simulink model "SSiWD_Lab2_blocks"  (R2015a)
settings: Solver=ode45  StartTime=0.0  StopTime=13  FixedStep=0.001  RelTol=1e-3
undefined symbols (not defined in the file or in its folder): sigbuilder_block
libraries: simulink x3, fuzblock x1
settings Model: Creator=Wojtek  LastModifiedBy=Szwank
settings DataIOCC: SignalLoggingSaveFormat=ModelDataLogs
settings DebuggingCC: SaveWithParameterizedLinksMsg=none  UnderspecifiedInitializationDetection=Classic  MergeDetectMultiDrivingBlocksExec=none  SolverPrmCheckMsg=warning  MultiTaskCondExecSysMsg=none  FcnCallInpInsideContextMsg=EnableAllAsWarning
settings GRTTargetCC: GeneratePreprocessorConditionals=Use local settings  CombineOutputUpdateFcns=off  GRTInterface=on

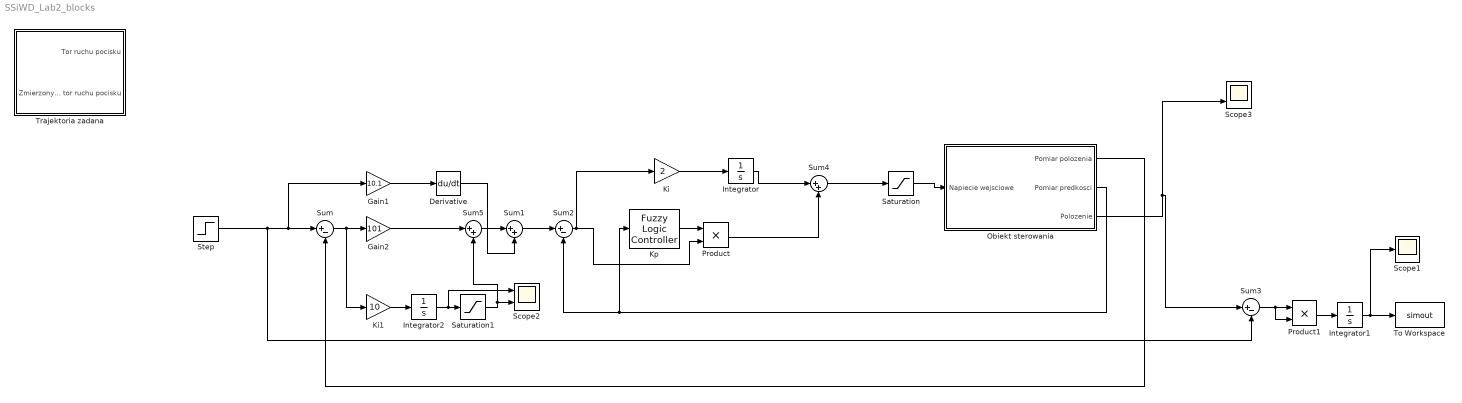
== system SSiWD_Lab2_blocks ==
  Derivative : Derivative
  Gain1 : Gain  Gain=10.1
  Gain2 : Gain  Gain=101
  Integrator : Integrator
  Integrator1 : Integrator  AbsoluteTolerance=0.001
  Integrator2 : Integrator
  Ki : Gain  Gain=2
  Ki1 : Gain  Gain=10
  Kp : fuzblock/Fuzzy Logic  Controller  fis=['regulator_prędkości.fis']
  Obiekt sterowania : Subsystem
  Product : Product
  Product1 : Product
  Saturation : Saturate  UpperLimit=50  LowerLimit=-50
  Saturation1 : Saturate  UpperLimit=70  LowerLimit=-70
  Scope1 : Scope
      settings: TimeRange=auto  MaxDataPoints=5000  SaveToWorkspace=off  YMin=-0.27846  YMax=2.50612  SampleTime=-1
  Scope2 : Scope  NumInputPorts=2
      settings: TimeRange=auto  MaxDataPoints=5000  SaveToWorkspace=off  SaveName=ScopeData2  YMin=-4.33652~-5  YMax=5.5637~5  SampleTime=-1
  Scope3 : Scope  NumInputPorts=2
      settings: TimeRange=auto  MaxDataPoints=5000  SaveToWorkspace=off  YMin=-1.96907~-5  YMax=4.71759~5  SampleTime=-1
  Step : Step  SampleTime=0.75
  Sum : Sum  Inputs=|+-
  Sum1 : Sum  Inputs=|++
  Sum2 : Sum  Inputs=|+-
  Sum3 : Sum  Inputs=|+-
  Sum4 : Sum  Inputs=|++
  Sum5 : Sum  Inputs=|++
  To Workspace : ToWorkspace  VariableName=simout  SampleTime=-1
  "Trajektoria zadana " : Subsystem
  wires:
  Obiekt sterowania/2(Pomiar predkosci) -> Kp/1, Sum2/2
  Obiekt sterowania/1(Pomiar polozenia) -> Sum/2
  Ki/1 -> Integrator/1
  Integrator/1 -> Sum4/1
  Saturation/1 -> Obiekt sterowania/1(Napiecie wejsciowe)
  Sum4/1 -> Saturation/1
  Product/1 -> Sum4/2
  Sum2/1 -> Ki/1, Product/2
  Derivative/1 -> Sum1/2
  Gain1/1 -> Derivative/1
  Kp/1 -> Product/1
  Integrator1/1 -> Scope1/1, To Workspace/1
  Sum/1 -> Ki1/1, Gain2/1
  Ki1/1 -> Integrator2/1
  Sum5/1 -> Sum1/1
  Gain2/1 -> Sum5/1
  Obiekt sterowania/3(Polozenie) -> Scope3/2, Sum3/1
  Sum1/1 -> Sum2/1
  Sum3/1 -> Product1/2, Product1/1
  Product1/1 -> Integrator1/1
  Integrator2/1 -> Scope2/1, Saturation1/1
  Saturation1/1 -> Scope2/2, Sum5/2
  Step/1 -> Sum3/2, Gain1/1, Sum/1

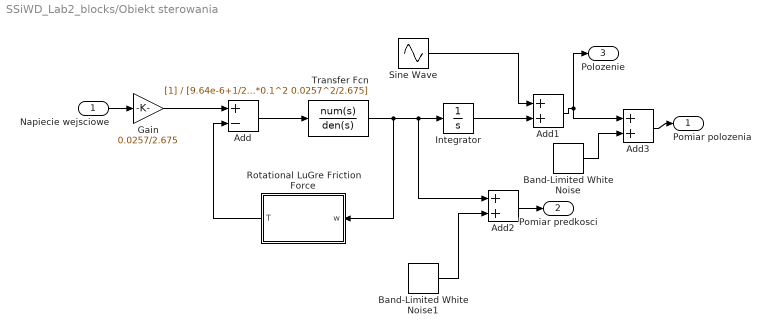
== system SSiWD_Lab2_blocks/Obiekt sterowania ==
  Napiecie wejsciowe : Inport
  Add : Sum  Inputs=+-
  Add1 : Sum
  Add2 : Sum
  Add3 : Sum
  Band-Limited White Noise : simulink/Sources/Band-Limited White Noise  Cov=[0.00001]  Ts=0.001  seed=[23341]
  Band-Limited White Noise1 : simulink/Sources/Band-Limited White Noise  Cov=[0.00001]  Ts=0.001  seed=[23341]
  Gain : Gain  Gain=0.0257/2.675
  Integrator : Integrator
  Rotational LuGre Friction Force : Subsystem  TreatAsAtomicUnit=on  mask(LuGre friction model){ro0=1.2, ro1=0.05, ro2=2.9e-6, Fc=0.77e-3, Fs=12e-3, Vs=0.09}
      mask prompts: Fc "Culomb force (Fc)"; Fs "Friction force (Fs)"; Vs "Striback velocity (Vs)"
      mask help:
      | The LuGre model is a dynamic friction model. The model is related to the bristle interpretation of friction. Friction is modeled as the average deflection force of elastic springs. When a tangential force is applied the bristles will deflect like springs. If the deflection is sufficiently large the bristles start to slip.
      |
      | The input signal is the velocity of the object. The output signal is the fristion force value.
      mask Help:
      | <!DOCTYPE html   PUBLIC "-//W3C//DTD HTML 4.01 Transitional//EN" "http://www.w3.org/TR/1999/REC-html401-19991224/loose.dtd">
      | <html lang="en"><head>
      | <meta http-equiv="Content-Type" content="text/html; charset=utf-8">
      | <title>About :: LuGre friction model</title>
      | <meta name="description" content="">
      | </head>
      | <body><a name="top_of_page"></a>
      | The LuGre model is a dynamic friction model. The model is related to
      | the bristle interpretation of friction. Friction is modeled as the average
      | deflection force of elastic springs. When a tangential force is applied the bristles
      | will deflect like springs. If the deflection is sufficiently large the bristles start
      | to slip. The average bristle deflection for a steady state motion is determined
      | by the velocity. It is lower at low velocities, which implies that the steady state
      | deflection decreases with increasing velocity. This models the phenomenon that
      | the surfaces are pushed apart by the lubricant, and models the Stribeck effect.
      | The model also includes rate dependent friction phenomena such as varying
      | break-away force and frictional lag.<sup><a href="#ref1">1</a></sup></p><p>More information about the model may be found in the labsheets.</p>
      | <hr><small>
      | <sup><a name="ref1"></a>1</sup> <b>Friction Models and Friction Compensation</b>. H. Olsson, K.J. &Aring;str&ouml;m, C. Canudas de Wit, M. G&auml;fvert, P. Lischinsky
      | </small>
      | <br />
      | <br />
      | <hr>
      | <center><small>Copyright&copy;2009
      | <a href="mailto:w.kurek@ely.pg.gda.pl">Wojciech Kurek</a>,
      | <a href="mailto:g.ewald@ely.pg.gda.pl">Grzegorz Ewald</a>
      | </small></center>
      | </body>
      | </html>
      mask Callback ro0:
      | if str2num(get_param(gcb, 'ro0')) <= 0
      |     error('ro0 is negative!')
      | end
      mask Callback ro1:
      | if str2num(get_param(gcb, 'ro1')) <= 0
      |     error('ro1 is negative!')
      | end
      mask Callback ro2:
      | if str2num(get_param(gcb, 'ro2')) <= 0
      |     error('ro2 is negative!')
      | end
      mask Callback Fc:
      | if str2num(get_param(gcb, 'Fs')) <= 0
      |     error('Culomb force is negative!')
      | end
      mask Callback Fs:
      | if str2num(get_param(gcb, 'Fs')) <= 0
      |     error('Friction force is negative!')
      | end
      mask Callback Vs:
      | if str2num(get_param(gcb, 'Vs')) <= 0
      |     error('Striback velocity is negative!')
      | end
      mask Display:
      | patch([0.1 0.1 0.9 0.9],[0.1 0.25 0.25 0.1],[0.8 0.8 0.8])
      | patch([0.1 0.1 0.9 0.9],[0.9 0.75 0.75 0.9],[0.8 0.8 0.8])
      | 
      | plot([0.12 0.12],[0.25 0.5])
      | plot([0.2 0.2],[0.25 0.5])
      | plot([0.4 0.4],[0.25 0.5])
      | plot([0.57 0.57],[0.25 0.5])
      | plot([0.67 0.67],[0.25 0.5])
      | plot([0.87 0.87],[0.25 0.5])
      | 
      | plot([0.17 0.18 0.2 0.23],[0.75 0.6 0.5 0.45])
      | plot([0.35 0.36 0.39 0.44],[0.75 0.6 0.5 0.48])
      | plot([0.62 0.64 0.68 0.72],[0.75 0.6 0.5 0.48])
      | plot([0.85 0.86 0.87 0.89],[0.75 0.6 0.5 0.48])
      | 
      | plot([0.15 0.15],[0.75 0.4])
      | plot([0.28 0.28],[0.75 0.4])
      | plot([0.55 0.55],[0.75 0.4])
      | plot([0.8 0.8],[0.75 0.4])
      | 
      | color('blue');
      | port_label('input',1,'\omega','texmode','on')
      | port_label('output',1,'T','texmode','on')
  Sine Wave : Sin  Amplitude=10  SampleTime=0
  Transfer Fcn : TransferFcn  Denominator=[9.64e-6+1/2*2.1*0.1^2 0.0257^2/2.675]
  Pomiar polozenia : Outport
  Pomiar predkosci : Outport  Port=2
  Polozenie : Outport  Port=3
  wires:
  Band-Limited White Noise/1 -> Add3/2
  Add3/1 -> Pomiar polozenia/1
  Add2/1 -> Pomiar predkosci/1
  Napiecie wejsciowe/1 -> Gain/1
  Add1/1 -> Add3/1, Polozenie/1
  Band-Limited White Noise1/1 -> Add2/2
  Integrator/1 -> Add1/2
  Sine Wave/1 -> Add1/1
  Add/1 -> Transfer Fcn/1
  Rotational LuGre Friction Force/1(T) -> Add/2
  Transfer Fcn/1 -> Add2/1, Integrator/1, Rotational LuGre Friction Force/1(w)
  Gain/1 -> Add/1

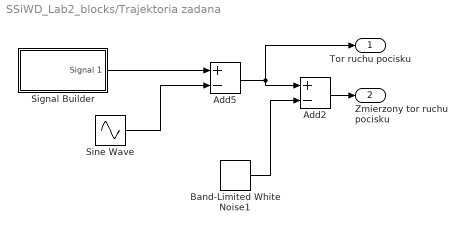
== system SSiWD_Lab2_blocks/Trajektoria zadana  ==
  Add2 : Sum  Inputs=+-
  Add5 : Sum  Inputs=+-
  Band-Limited White Noise1 : simulink/Sources/Band-Limited White Noise  Cov=[0.00001]  Ts=0.001  seed=[23341]
  Signal Builder : Subsystem  Tag=STV Subsys  LoadFcn=sigbuilder_block('load');  StartFcn=sigbuilder_block('start');  StopFcn=sigbuilder_block('stop');  ClipboardFcn=sigbuilder_block('clipboard');  mask(Sigbuilder block){}
      mask help: Simulink:masks:SigbuilderBlock_MD
      mask init:
      | if ~strcmp(get_param(bdroot(gcbh),'SimulationStatus'),'stopped') tuvar = sigbuilder_block('maskInit'); end
      settings: CopyFcn=sigbuilder_block('copy');  DeleteFcn=sigbuilder_block('delete');  ModelCloseFcn=sigbuilder_block('modelClose');  PreSaveFcn=sigbuilder_block('preSave');  PauseFcn=sigbuilder_block('pause');  ContinueFcn=sigbuilder_block('continue');  NameChangeFcn=sigbuilder_block('namechange');  OpenFcn=sigbuilder_block('open',[437.6 199.2 550.4 400 ]);  CloseFcn=sigbuilder_block('close');
      mask Display: plot(0, 0, 100, 100,[2, 2, 32, 32, 2], [68, 8, 8, 68, 68],[32, 2], [38, 38], [32, 19, 2],[53, 60, 44], [32, 17, 17, 2],[16, 16, 31, 31]);txt = getActiveGroup(gcbh);text(2, 100, txt,'verticalAlignment', 'top');
  Sine Wave : Sin  Amplitude=2  SampleTime=0
  Tor ruchu pocisku : Outport
  Zmierzony tor ruchu pocisku : Outport  Port=2
  wires:
  Add2/1 -> Zmierzony tor ruchu pocisku/1
  Sine Wave/1 -> Add5/2
  Signal Builder/1(Signal 1) -> Add5/1
  Add5/1 -> Tor ruchu pocisku/1, Add2/1
  Band-Limited White Noise1/1 -> Add2/2

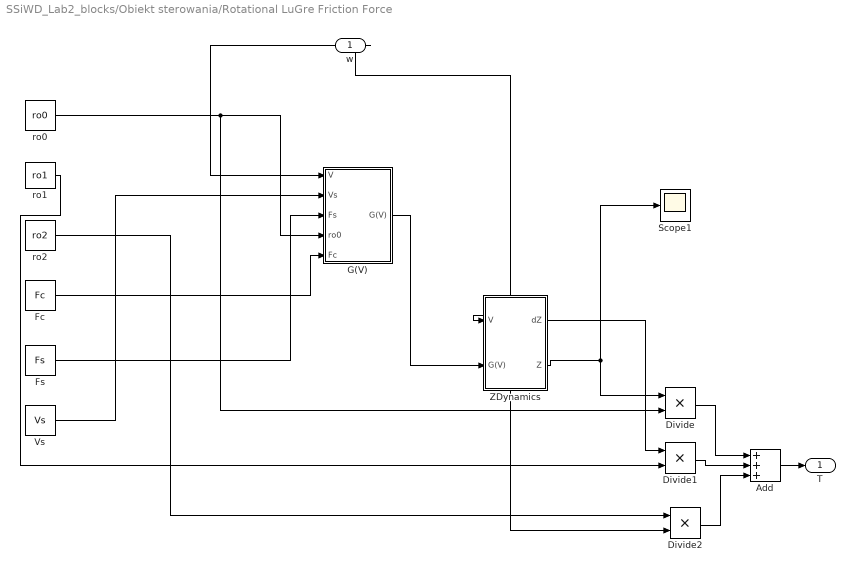
== system SSiWD_Lab2_blocks/Obiekt sterowania/Rotational LuGre Friction Force ==
  w : Inport
  Add : Sum  Inputs=+++
  Divide : Product  Inputs=**
  Divide1 : Product  Inputs=**
  Divide2 : Product  Inputs=**
  Fc : Constant  Value=Fc
  Fs : Constant  Value=Fs
  G(V) : Subsystem
  Scope1 : Scope
      settings: TimeRange=auto  MaxDataPoints=5000  SaveToWorkspace=off  SaveName=ScopeData3  YMin=-1  YMax=1  SampleTime=-1
  Vs : Constant  Value=Vs
  ZDynamics : Subsystem
  ro0 : Constant  Value=ro0
  ro1 : Constant  Value=ro1
  ro2 : Constant  Value=ro2
  T : Outport
  wires:
  Add/1 -> T/1
  Divide2/1 -> Add/3
  Divide1/1 -> Add/2
  Divide/1 -> Add/1
  ro2/1 -> Divide2/1
  ro1/1 -> Divide1/2
  ZDynamics/1(dZ) -> Divide1/1
  ZDynamics/2(Z) -> Scope1/1, Divide/1
  G(V)/1(G(V)) -> ZDynamics/2(G(V))
  ro0/1 -> Divide/2, G(V)/4(ro0)
  Fc/1 -> G(V)/5(Fc)
  Fs/1 -> G(V)/3(Fs)
  Vs/1 -> G(V)/2(Vs)
  w/1 -> G(V)/1(V), ZDynamics/1(V), Divide2/2

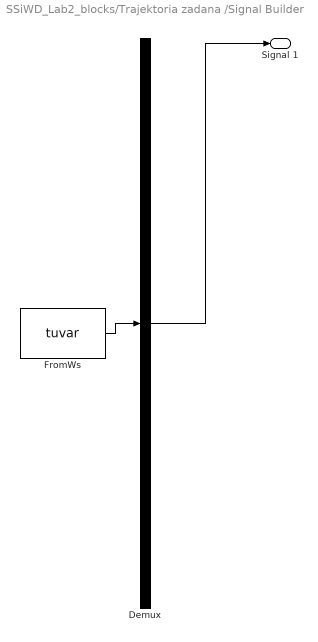
== system SSiWD_Lab2_blocks/Trajektoria zadana /Signal Builder ==
  Demux : Demux  Tag=STV Demux  Outputs=1
  FromWs : FromWorkspace  Tag=STV FromWs  VariableName=tuvar  SampleTime=0
      SigBuilderData=|
      | common.afterFinalStr = 'Extrapolate'
      | common.sampleTime = 0
      | dataSet.timeRange = [0 20]
      | dataSet.name = 'Group 1'
      | sbobj.Groups.Name = 'Group 1'
      | sbobj.Groups.Signals.Name = 'Signal 1'
      | sbobj.Groups.Signals.XData = [0 4 6 9 13.5 15.4 20]
      | sbobj.Groups.Signals.YData = [30 31 32 24 7 1.2 0]
      | sbobj.Groups.TimeRange = [0 20]
  Signal 1 : Outport  Tag=STV Outport
  wires:
  Demux/1 -> Signal 1/1
  FromWs/1 -> Demux/1

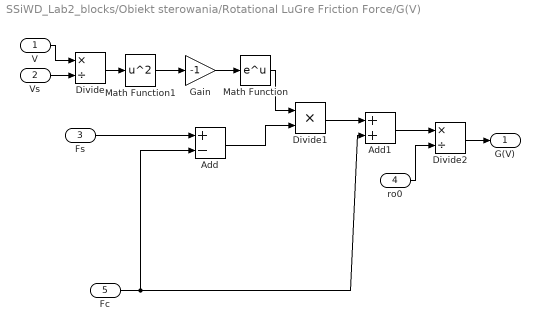
== system SSiWD_Lab2_blocks/Obiekt sterowania/Rotational LuGre Friction Force/G(V) ==
  V : Inport
  Vs : Inport  Port=2
  Fs : Inport  Port=3
  ro0 : Inport  Port=4
  Fc : Inport  Port=5
  Add : Sum  Inputs=+-
  Add1 : Sum
  Divide : Product  Inputs=*/
  Divide1 : Product  Inputs=**
  Divide2 : Product  Inputs=*/
  Gain : Gain  Gain=-1
  Math Function : Math  SaturateOnIntegerOverflow=on
  Math Function1 : Math  Operator=square  SaturateOnIntegerOverflow=on
  G(V) : Outport
  wires:
  Math Function/1 -> Divide1/1
  Gain/1 -> Math Function/1
  Math Function1/1 -> Gain/1
  ro0/1 -> Divide2/2
  Divide2/1 -> G(V)/1
  Fs/1 -> Add/1
  Vs/1 -> Divide/2
  V/1 -> Divide/1
  Add1/1 -> Divide2/1
  Divide1/1 -> Add1/1
  Add/1 -> Divide1/2
  Fc/1 -> Add/2, Add1/2
  Divide/1 -> Math Function1/1

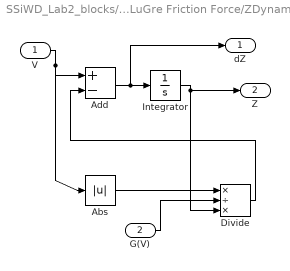
== system SSiWD_Lab2_blocks/Obiekt sterowania/Rotational LuGre Friction Force/ZDynamics ==
  V : Inport
  G(V) : Inport  Port=2
  Abs : Abs
  Add : Sum  Inputs=+-
  Divide : Product  Inputs=*/*
  Integrator : Integrator
  dZ : Outport
  Z : Outport  Port=2
  wires:
  G(V)/1 -> Divide/2
  V/1 -> Abs/1, Add/1
  Divide/1 -> Add/2
  Integrator/1 -> Z/1, Divide/3
  Abs/1 -> Divide/1
  Add/1 -> dZ/1, Integrator/1
